simulink model "kalmanlinear"  (R2019b)
settings: Solver=VariableStepAuto  StartTime=0.0  StopTime=25  RelTol=1e-3
undefined symbols (not defined in the file or in its folder): Continuous, Time
libraries: ctrlSharedLib x3
settings Model: Creator=Bekircan Keceoglu  LastModifiedBy=Bekircan Keceoglu

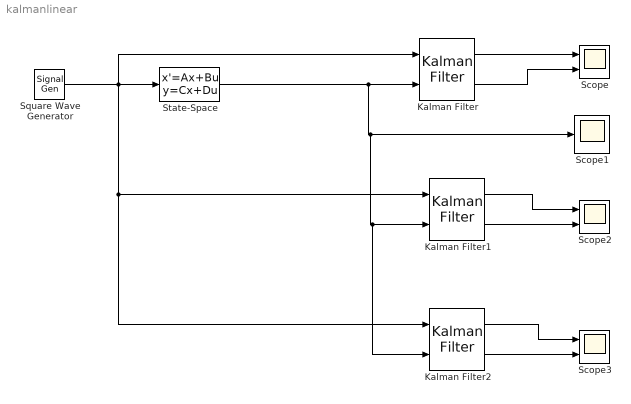
== system kalmanlinear ==
  Kalman Filter : ctrlSharedLib/Kalman Filter  TimeDomain=Continuous-Time  UseCurrentEstimator=on  ModelSource=Individual A, B, C, D matrices  ModelSourceVariable=ss(0.95,1,1,0,1)  A=[-1 -0.01; 1 0]  B=[1;0]  C=[0 1]  D=[0]  NumberOfStates=1  NumberOfInputs=1  NumberOfOutputs=1  InitialEstimateSource=Dialog  X0=0  P0=10  UseK=off  UseGH=off  NumberOfProcessNoiseInputs=1  G=1  TimeInvariantG=on  H=0  TimeInvariantH=on  Q=1  TimeInvariantQ=on  R=1  TimeInvariantR=on  N=0  TimeInvariantN=on  AddInputPort=on  AddEnablePort=off  OutputEstimatedY=on  OutputP=off  Ts=-1
      settings: SourceProductBaseCode=CT
  Kalman Filter1 : ctrlSharedLib/Kalman Filter  TimeDomain=Continuous-Time  UseCurrentEstimator=on  ModelSource=Individual A, B, C, D matrices  ModelSourceVariable=ss(0.95,1,1,0,1)  A=[-1 -0.01; 1 0]  B=[1;0]  C=[0 1]  D=[0]  NumberOfStates=1  NumberOfInputs=1  NumberOfOutputs=1  InitialEstimateSource=Dialog  X0=0  P0=10  UseK=off  UseGH=off  NumberOfProcessNoiseInputs=1  G=1  TimeInvariantG=on  H=0  TimeInvariantH=on  Q=10  TimeInvariantQ=on  R=0.1  TimeInvariantR=on  N=0  TimeInvariantN=on  AddInputPort=on  AddEnablePort=off  OutputEstimatedY=on  OutputP=off  Ts=-1
      settings: SourceProductBaseCode=CT
  Kalman Filter2 : ctrlSharedLib/Kalman Filter  TimeDomain=Continuous-Time  UseCurrentEstimator=on  ModelSource=Individual A, B, C, D matrices  ModelSourceVariable=ss(0.95,1,1,0,1)  A=[-1 -0.01; 1 0]  B=[1;0]  C=[0 1]  D=[0]  NumberOfStates=1  NumberOfInputs=1  NumberOfOutputs=1  InitialEstimateSource=Dialog  X0=0  P0=10  UseK=off  UseGH=off  NumberOfProcessNoiseInputs=1  G=1  TimeInvariantG=on  H=0  TimeInvariantH=on  Q=0.1  TimeInvariantQ=on  R=10  TimeInvariantR=on  N=0  TimeInvariantN=on  AddInputPort=on  AddEnablePort=off  OutputEstimatedY=on  OutputP=off  Ts=-1
      settings: SourceProductBaseCode=CT
  Scope : Scope  NumInputPorts=2
  Scope1 : Scope
  Scope2 : Scope  NumInputPorts=2
  Scope3 : Scope  NumInputPorts=2
  Square Wave Generator : SignalGenerator  WaveForm=square  Units=rad/sec
  State-Space : StateSpace  A=[-1 -0.01; 1 0]  B=[1; 0]  C=[0 1]  D=[0]  InitialCondition=[0 0]
  wires:
  Square Wave Generator/1 -> Kalman Filter2/1, Kalman Filter1/1, Kalman Filter/1, State-Space/1
  State-Space/1 -> Kalman Filter2/2, Kalman Filter1/2, Scope1/1, Kalman Filter/2
  Kalman Filter/2 -> Scope/2
  Kalman Filter2/2 -> Scope3/2
  Kalman Filter2/1 -> Scope3/1
  Kalman Filter1/2 -> Scope2/2
  Kalman Filter1/1 -> Scope2/1
  Kalman Filter/1 -> Scope/1
